simulink model "Landing_Gear_Suspension_system"  (R2021a)
settings: Solver=FixedStepAuto  StartTime=0.0  StopTime=100  FixedStep=0.001  RelTol=1e-3
model workspace: external: MATLAB File D:\Aerospace\UDC Control and Simulation Recruitment Task\Task I - Physical Modeling\Physical_Modeling_Parameters.m (data not in the file)
values from neighbouring files (symbols this model uses):
  B1 = 350    [Physical_Modeling_Parameters.m]
  B2 = 15020    [Physical_Modeling_Parameters.m]
  K1 = 80000    [Physical_Modeling_Parameters.m]
  K2 = 500000    [Physical_Modeling_Parameters.m]
  M1 = 2500    [Physical_Modeling_Parameters.m]
  M2 = 320    [Physical_Modeling_Parameters.m]
settings Model: OrderedModelArguments=off  Creator=aabdu  LastModifiedBy=aabdu

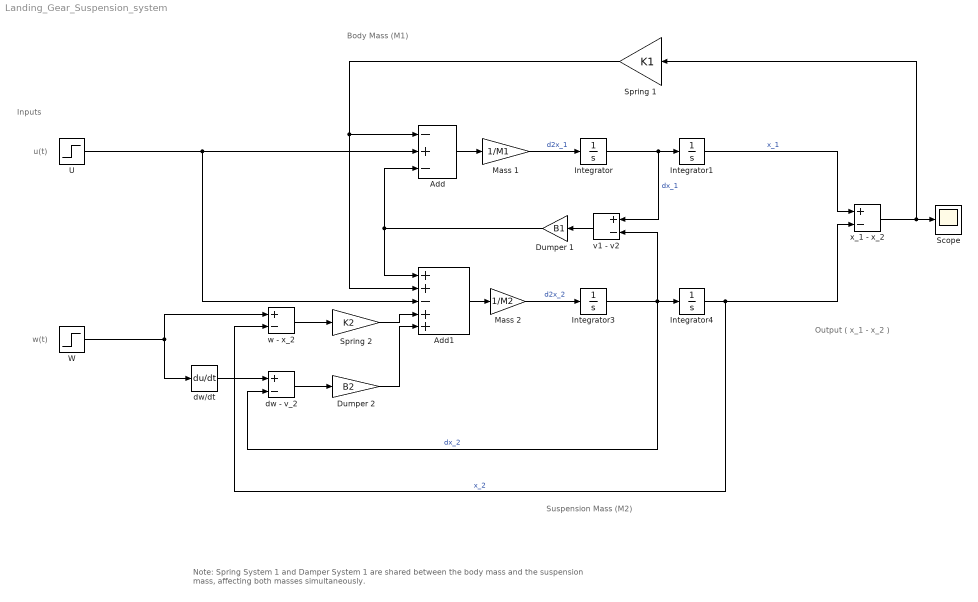
== system Landing_Gear_Suspension_system ==
  note: Note: Spring System 1 and Damper System 1 are shared between the body mass and the suspension mass, affecting both masses simultaneously.
  note: Body Mass (M1)
  note: Inputs
  note: u(t)
  note: Output ( x_1 - x_2 )
  note: w(t)
  note: Suspension Mass (M2)
  Add : Sum  Inputs=-+-
  Add1 : Sum  Inputs=++-++
  Dumper 1 : Gain  Gain=B1
  Dumper 2 : Gain  Gain=B2
  Integrator{,1,3..4} (4 alike) : Integrator
  Mass 1 : Gain  Gain=1/M1
  Mass 2 : Gain  Gain=1/M2
  Scope : Scope
  Spring 1 : Gain  Gain=K1
  Spring 2 : Gain  Gain=K2
  U : Step  Description=U  Time=0  After=0  SampleTime=0
  W : Step  Time=5  After=-0.1  SampleTime=0
  dw - v_2 : Sum  Inputs=+-
  dw/dt : Derivative
  v1 - v2 : Sum  Inputs=+-
  w - x_2 : Sum  Inputs=+-
  x_1 - x_2 : Sum  Inputs=+-
  wires:
  Integrator/1 -> v1 - v2/1, Integrator1/1  "dx_1"
  Integrator1/1 -> x_1 - x_2/1  "x_1"
  Integrator3/1 -> dw - v_2/2, v1 - v2/2, Integrator4/1  "dx_2"
  Integrator4/1 -> w - x_2/2, x_1 - x_2/2  "x_2"
  Mass 2/1 -> Integrator3/1  "d2x_2"
  x_1 - x_2/1 -> Spring 1/1, Scope/1
  Add/1 -> Mass 1/1
  Mass 1/1 -> Integrator/1  "d2x_1"
  Add1/1 -> Mass 2/1
  U/1 -> Add1/3, Add/2
  Spring 1/1 -> Add1/2, Add/1
  v1 - v2/1 -> Dumper 1/1
  Dumper 1/1 -> Add1/1, Add/3
  dw/dt/1 -> dw - v_2/1
  W/1 -> w - x_2/1, dw/dt/1
  w - x_2/1 -> Spring 2/1
  Spring 2/1 -> Add1/4
  dw - v_2/1 -> Dumper 2/1
  Dumper 2/1 -> Add1/5
